simulink model "car3"  (R2016a)
settings: Solver=ode5  StartTime=0.0  StopTime=10  FixedStep=0.001  RelTol=1e-3
values from neighbouring files (symbols this model uses):
  E = eye(8)    [car.m]    (also in car_m.m = eye(2))
  LK1 = -LK1    [car.m]    (also in car_m.m = [-1 0;0 -1]')
  v0 = [1 1 2 1 1 1 1 1]'    [car.m]    (also in car_m.m = [1 1]')
  x0 = [1 3 2 1 3 2 4 5]'    [car.m]    (also in car_m.m = [0 0]')
  xd = [10 10]    [car_m.m]
settings Model: Creator=richa  LastModifiedBy=richa

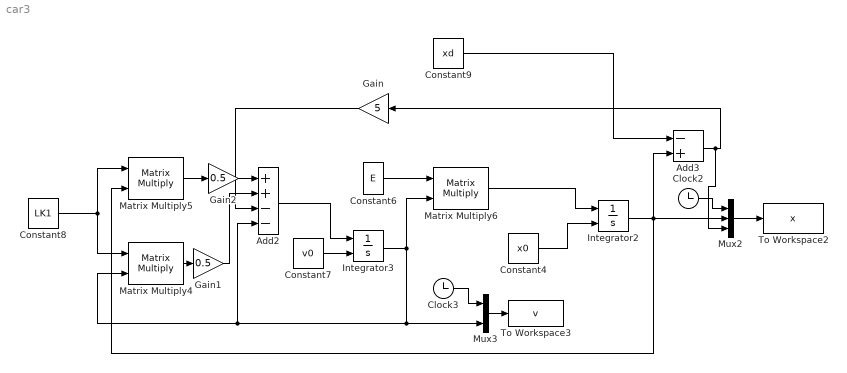
== system car3 ==
  Add2 : Sum  Inputs=++--
  Add3 : Sum  Inputs=-+
  Clock2 : Clock
  Clock3 : Clock
  Constant4 : Constant  Value=x0
  Constant6 : Constant  Value=E
  Constant7 : Constant  Value=v0
  Constant8 : Constant  Value=LK1
  Constant9 : Constant  Value=xd
  Gain : Gain  Gain=5
  Gain1 : Gain  Gain=0.5
  Gain2 : Gain  Gain=0.5
  Integrator2 : Integrator  InitialConditionSource=external
  Integrator3 : Integrator  InitialConditionSource=external
  Matrix Multiply4 : Product  Multiplication=Matrix(*)
  Matrix Multiply5 : Product  Multiplication=Matrix(*)
  Matrix Multiply6 : Product  Multiplication=Matrix(*)
  Mux2 : Mux  Inputs=3
  Mux3 : Mux  Inputs=2
  To Workspace2 : ToWorkspace  VariableName=x  SampleTime=-1
  To Workspace3 : ToWorkspace  VariableName=v  SampleTime=-1
  wires:
  Constant4/1 -> Integrator2/2
  Mux2/1 -> To Workspace2/1
  Clock2/1 -> Mux2/1
  Constant7/1 -> Integrator3/2
  Constant8/1 -> Matrix Multiply4/1, Matrix Multiply5/1
  Mux3/1 -> To Workspace3/1
  Clock3/1 -> Mux3/1
  Add2/1 -> Integrator3/1
  Constant6/1 -> Matrix Multiply6/1
  Matrix Multiply6/1 -> Integrator2/1
  Add3/1 -> Mux2/3, Gain/1
  Integrator2/1 -> Add3/2, Matrix Multiply5/2, Mux2/2
  Integrator3/1 -> Matrix Multiply6/2, Add2/4, Matrix Multiply4/2, Mux3/2
  Constant9/1 -> Add3/1
  Gain/1 -> Add2/3
  Matrix Multiply4/1 -> Gain1/1
  Gain1/1 -> Add2/2
  Matrix Multiply5/1 -> Gain2/1
  Gain2/1 -> Add2/1
